simulink model "ex7"  (Simulink 6.3)
settings: Solver=VariableStepDiscrete  StartTime=0.0  StopTime=1  RelTol=1e-3
values from neighbouring files (symbols this model uses):
  BER = ber(ii)    [ex7sim.m]    (also in ex9sim.m)
undefined symbols (not defined in the file or in its folder): rsgenpoly
libraries: dspobslib x5, commblkcod2 x2, commchan3 x1, commsink2 x1, commrandsrc2 x1
settings Model: LastModifiedBy=lxy  StrictBusMsg=None
settings OptimizationCC: InlineInvariantSignals=on

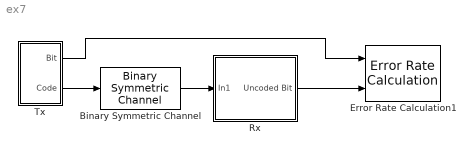
== system ex7 ==
  Binary Symmetric Channel : commchan3/Binary Symmetric Channel  P=BER  s=71  E=off  outDtype=double
  Error Rate Calculation1 : commsink2/Error Rate Calculation  N=0  st_delay=0  cp_mode=Entire frame  subframe=[]  PMode=Workspace  WsName=BER1  RsMode2=off  stop=off  numErr=100  maxBits=1e6
  Rx : Subsystem
  Tx : Subsystem
  wires:
  Binary Symmetric Channel/1 -> Rx/1(In1)
  Rx/1(Uncoded Bit) -> Error Rate Calculation1/2
  Tx/1(Bit) -> Error Rate Calculation1/1
  Tx/2(Code) -> Binary Symmetric Channel/1

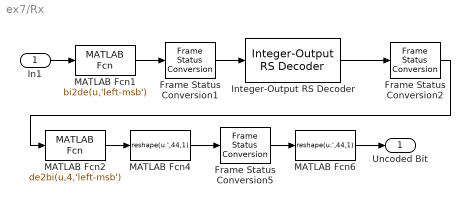
== system ex7/Rx ==
  In1 : Inport
  Frame Status Conversion1 : dspobslib/Frame Status Conversion  growRefPort=off  outframe=Frame-based
  Frame Status Conversion2 : dspobslib/Frame Status Conversion  growRefPort=off  outframe=Sample-based
  Frame Status Conversion5 : dspobslib/Frame Status Conversion  growRefPort=off  outframe=Frame-based
  Integer-Output RS Decoder : commblkcod2/Integer-Output RS Decoder  n=15  k=11  specPrimPoly=off  primPoly=[1 0 1 1]  specGenPoly=off  genPoly=rsgenpoly(7,3)  showNumErr=off
  MATLAB Fcn1 : MATLABFcn  MATLABFcn=bi2de(u,'left-msb')
  MATLAB Fcn2 : MATLABFcn  MATLABFcn=de2bi(u,4,'left-msb')  Output1D=off
  MATLAB Fcn4 : MATLABFcn  MATLABFcn=reshape(u.',44,1)  OutputSignalType=real  Output1D=off
  MATLAB Fcn6 : MATLABFcn  MATLABFcn=reshape(u.',44,1)  OutputSignalType=real  Output1D=off
  Uncoded Bit : Outport
  wires:
  MATLAB Fcn1/1 -> Frame Status Conversion1/1
  Frame Status Conversion1/1 -> Integer-Output RS Decoder/1
  Integer-Output RS Decoder/1 -> Frame Status Conversion2/1
  MATLAB Fcn2/1 -> MATLAB Fcn4/1
  MATLAB Fcn4/1 -> Frame Status Conversion5/1
  Frame Status Conversion5/1 -> MATLAB Fcn6/1
  MATLAB Fcn6/1 -> Uncoded Bit/1
  In1/1 -> MATLAB Fcn1/1
  Frame Status Conversion2/1 -> MATLAB Fcn2/1

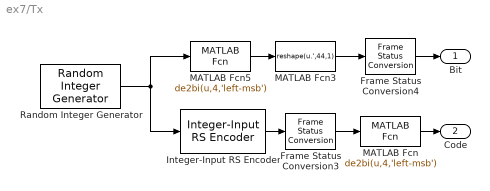
== system ex7/Tx ==
  Frame Status Conversion3 : dspobslib/Frame Status Conversion  growRefPort=off  outframe=Sample-based
  Frame Status Conversion4 : dspobslib/Frame Status Conversion  growRefPort=off  outframe=Frame-based
  Integer-Input RS Encoder : commblkcod2/Integer-Input RS Encoder  n=15  k=11  specPrimPoly=off  primPoly=[1 0 1 1]  specGenPoly=off  genPoly=rsgenpoly(7,3)
  MATLAB Fcn : MATLABFcn  MATLABFcn=de2bi(u,4,'left-msb')  Output1D=off
  MATLAB Fcn3 : MATLABFcn  MATLABFcn=reshape(u.',44,1)  OutputSignalType=real  Output1D=off
  MATLAB Fcn5 : MATLABFcn  MATLABFcn=de2bi(u,4,'left-msb')  Output1D=off
  Random Integer Generator : commrandsrc2/Random Integer Generator  mul=16  seed=37  Ts=1/110000  frameBased=on  sampPerFrame=11  orient=off  outDataType=double
  Bit : Outport
  Code : Outport  Port=2
  wires:
  Integer-Input RS Encoder/1 -> Frame Status Conversion3/1
  Frame Status Conversion3/1 -> MATLAB Fcn/1
  MATLAB Fcn3/1 -> Frame Status Conversion4/1
  MATLAB Fcn5/1 -> MATLAB Fcn3/1
  Frame Status Conversion4/1 -> Bit/1
  MATLAB Fcn/1 -> Code/1
  Random Integer Generator/1 -> MATLAB Fcn5/1, Integer-Input RS Encoder/1
